simulink subsystem "Vehicle_Model_Simplified"  (R2023b)
settings: Solver=VariableStepAuto  StartTime=0.0  StopTime=10.0  RelTol=1e-3
values from neighbouring files (symbols this model uses):
  phi = 45    [Data_Parse_Events.m]
  theta = Digital_Signals.Corner_Dynamics_Sensors.theta.Data    [Yaw_Tables.m]    (also in compute_axis_transformation.m = acos(dot(XYZs,XYZv)/(norm(XYZv)^2)); create_yaw_table.m = acos(dot(XYZs,XYZv)/(norm(XYZv)^2)))
undefined symbols (not defined in the file or in its folder): chassis, dZ, F0z, powertrain, psi, sim, suspension, VEH, X, Xdot, Y, Ydot, Z, Zdot
libraries: vehdynlibtire x10, vehdynlibsuspension x8, autolibutils x5, sharedtransform x5, shared6dof x2, dspstat3 x1, vehdynlibeom x1, vehdynlibtirecommon x1
(part 2 of 6)

== system Vehicle_Model_Simplified/Suspension/MacPherson Suspension ==
  Wheel : Inport
  Steering : Inport  Port=2
  Vehicle : Inport  Port=3
  Bus Creator1 : BusCreator  Inputs=6
  Bus Creator2 : BusCreator  Inputs=2
  Bus Creator3 : BusCreator  Inputs=2
  Bus Creator4 : BusCreator  Inputs=6
  Bus Selector : BusSelector  OutputSignals=z,Re,zdot,Fx,Fy,M
  Bus Selector1 : BusSelector  OutputSignals=P,V
  Bus Selector2 : BusSelector  OutputSignals=SuspFrame.z
  Selector1 : Selector  NumberOfDimensions=2  IndexOptions=Index vector (dialog),Select all  Indices=1,1  OutputSizes=1,1
  Selector2 : Selector  NumberOfDimensions=2  IndexOptions=Index vector (dialog),Select all  Indices=2,1  OutputSizes=1,1
  Steer Rate Adapter : Subsystem
  Steering Adapter : Subsystem
  Terminator : Terminator
  Terminator1 : Terminator
  Vehicle Adapter : Subsystem
  Wheel  Adapter : Subsystem
  Wheel1 : InportShadow
  independent Suspensions - MacPherson : vehdynlibsuspension/Independent Suspension - MacPherson  ActiveDampEn=off  NumAxl=2  NumWhlsByAxl=[2 2]  StrgEnByAxl=[1 0]  AntiSwayEnByAxl=[1 0]  WhlNumVec="[1  2  1  2]"  AxleNumVec="[1  1  2  2]"  SuspTypesByAxle="[1  1]"  SuspImage=suspmacp.png  IdealSuspEn=on  IdealSuspAxles="[1  2]"  Kz=Kz  F0z=F0z  Cz=Cz  Hmax=Hmax  f_act_susp_cz=[10000 10000;10000 10000]  f_act_susp_duty_bpt=[0 1]  f_act_susp_zdot_bpt=[-1 1]  Toe=0.  RollStrgSlp=0.  ToeStrgSlp=0.  Caster=0.  CasterHslp=0.  CasterStrgSlp=0.  Camber=0.  CamberHslp=0.  CamberStrgSlp=0.  StrgHgtSlp=0.1432  MappedSuspEn=off  MappedSuspAxles="[1  2]"  f_susp_axl_bp=[1 2]  f_susp_dz_bp=[-0.15 -0.14 -0.13 -0.12 -0.11 -0.10 -0.09 -0.08 -0.07 -0.06 -0.05 -0.04 -0.03 -0.02 -0.01 0.00 0.01 0.02 0.03 0.04 0.05 0.06 0.07 0.08 0.09 0.10 0.11 0.12 0.13 0.14 0.15]  f_susp_dzdot_bp=[-0.15 -0.14 -0.13 -0.12 -0.11 -0.10 -0.09 -0.08 -0.07 -0.06 -0.05 -0.04 -0.03 -0.02 -0.01 0.00 0.01 0.02 0.03 0.04 0.05 0.06 0.07 0.08 0.09 0.10 0.11 0.12 0.13 0.14 0.15]  f_susp_fmz=zeros(31,31,61,2,4)  f_susp_geom=zeros(31,61,2,3)  f_susp_strgdelta_bp=[-30,-29,-28,-27,-26,-25,-24,-23,-22,-21,-20,-19,-18,-17,-16,-15,-14,-13,-12,-11,-10,-9,-8,-7,-6,-5,-4,-3,-2,-1,0,1,2,3,4,5,6,7,8,9,10,11,12,13,14,15,16,17,18,19,20,21,22,23,24,25,26,27,28,29,30]  AntiSwayR=0.2  AntiSwayNtrlAng=0.5236  AntiSwayTrsK=8e+02
  Suspension : Outport  VectorParamsAs1DForOutWhenUnconnected=off
  wires:
  Bus Creator3/1 -> Suspension/1
  Bus Creator1/1 -> Bus Creator3/2  "Whl"
  Bus Selector1/2 -> independent Suspensions - MacPherson/8  "<V>"
  Bus Selector/6 -> independent Suspensions - MacPherson/6  "<M>"
  Bus Selector/5 -> independent Suspensions - MacPherson/5  "<Fy>"
  Steering/1 -> Steering Adapter/1(Steer)
  Bus Selector/3 -> independent Suspensions - MacPherson/3  "<zdot>"
  Bus Selector/4 -> independent Suspensions - MacPherson/4  "<Fx>"
  Vehicle/1 -> Vehicle Adapter/1(Veh), Steer Rate Adapter/1(Veh)
  Vehicle Adapter/1(VehSusp) -> Bus Selector1/1
  independent Suspensions - MacPherson/3 -> Bus Creator2/2  "M"
  Wheel  Adapter/2(WhlFy) -> Bus Creator4/2  "Fy"
  Wheel  Adapter/1(WhlFx) -> Bus Creator4/1  "Fx"
  Wheel/1 -> Wheel  Adapter/1(Wheels)
  Wheel  Adapter/3(z) -> Bus Creator4/3
  Wheel  Adapter/4(zdot) -> Bus Creator4/4
  Wheel  Adapter/5(M) -> Bus Creator4/5  "M"
  Wheel  Adapter/6(Re) -> Bus Creator4/6
  Bus Selector/2 -> independent Suspensions - MacPherson/2  "<Re>"
  Selector1/1 -> Bus Creator1/2  "xdot"
  Selector2/1 -> Bus Creator1/3  "ydot"
  Bus Selector1/1 -> independent Suspensions - MacPherson/7  "<P>"
  Bus Selector/1 -> independent Suspensions - MacPherson/1  "<z>"
  independent Suspensions - MacPherson/4 -> Bus Creator1/1  "F"
  independent Suspensions - MacPherson/6 -> Bus Creator1/4  "Ang"
  Vehicle Adapter/2(VehVbody) -> Selector1/1, Selector2/1  "V"
  independent Suspensions - MacPherson/2 -> Bus Creator2/1  "F"
  Bus Creator2/1 -> Bus Creator3/1  "Veh"
  Bus Creator4/1 -> Bus Selector/1
  Steer Rate Adapter/1(AngVel) -> Bus Creator1/6  "AngVel"
  Steering Adapter/1(StrgAng) -> independent Suspensions - MacPherson/9
  independent Suspensions - MacPherson/1 -> Terminator/1
  independent Suspensions - MacPherson/5 -> Terminator1/1  "V"
  Bus Selector2/1 -> Bus Creator1/5  "<z>"
  Wheel1/1 -> Bus Selector2/1

== system Vehicle_Model_Simplified/Suspension/Mapped Suspension ==
  Wheel : Inport
  Steering : Inport  Port=2
  Vehicle : Inport  Port=3
  Bus Creator1 : BusCreator  Inputs=6
  Bus Creator2 : BusCreator  Inputs=2
  Bus Creator3 : BusCreator  Inputs=2
  Bus Creator4 : BusCreator  Inputs=6
  Bus Selector : BusSelector  OutputSignals=z,Re,zdot,Fx,Fy,M
  Bus Selector1 : BusSelector  OutputSignals=P,V
  Bus Selector2 : BusSelector  OutputSignals=SuspFrame.z
  Independent Suspension - Mapped : vehdynlibsuspension/Independent Suspension - Mapped  NumAxl=2  NumWhlsByAxl=[2 2]  StrgEnByAxl=[1 0]  AntiSwayEnByAxl=[1 1]  WhlNumVec="[1  2  1  2]"  AxleNumVec="[1  1  2  2]"  SuspTypesByAxle="[2  2]"  SuspImage=suspindmap.png  IdealSuspEn=off  IdealSuspAxles="[1  2]"  Kz=64370  F0z=9810  Cz=10000  Hmax=0.5  Toe=2  RollStrgSlp=-13  ToeStrgSlp=0.01  Caster=4  CasterHslp=-13  CasterStrgSlp=0.01  Camber=4  CamberHslp=-13  CamberStrgSlp=0.01  StrgHgtSlp=0.0025  MappedSuspEn=on  MappedSuspAxles="[1  2]"  f_susp_axl_bp=[1 2]  f_susp_dz_bp=f_susp_dz_bp  f_susp_dzdot_bp=f_susp_dzdot_bp  f_susp_fmz=f_susp_fmz  f_susp_geom=f_susp_geom  f_susp_strgdelta_bp=f_susp_strgdelta_bp  NDFLookupOutType=1:4  NDGLookupOutType=1:3  AntiSwayR=0.2  AntiSwayNtrlAng=0.5236  AntiSwayTrsK=8e2
      link override For each track and axle combination calculate suspension forces and moments/Suspension/Suspension Angle Calculations: OverrideUsingVariant=MappedSteeringEnabled
      link override For each track and axle combination calculate suspension forces and moments/Suspension/Z axis suspension characteristic: OverrideUsingVariant=MappedSuspension
  Reshape1 : Reshape  OutputDimensionality=Row vector (2-D)
  Selector : Selector  IndexOptions=Index vector (dialog)  Indices=[1 2]  OutputSizes=1
  Selector1 : Selector  NumberOfDimensions=2  IndexOptions=Index vector (dialog),Select all  Indices=1,1  OutputSizes=1,1
  Selector2 : Selector  NumberOfDimensions=2  IndexOptions=Index vector (dialog),Select all  Indices=2,1  OutputSizes=1,1
  Steer Rate Adapter : Subsystem
  Terminator : Terminator
  Terminator1 : Terminator
  Vehicle Adapter : Subsystem
  Wheel  Adapter : Subsystem
  Wheel1 : InportShadow
  Suspension : Outport  VectorParamsAs1DForOutWhenUnconnected=off
  wires:
  Independent Suspension - Mapped/1 -> Terminator/1
  Reshape1/1 -> Independent Suspension - Mapped/9
  Bus Selector/5 -> Independent Suspension - Mapped/5  "<Fy>"
  Bus Selector/2 -> Independent Suspension - Mapped/2  "<Re>"
  Bus Selector1/2 -> Independent Suspension - Mapped/8  "<V>"
  Bus Selector/4 -> Independent Suspension - Mapped/4  "<Fx>"
  Wheel  Adapter/5(M) -> Bus Creator4/5
  Bus Selector/6 -> Independent Suspension - Mapped/6  "<M>"
  Wheel  Adapter/4(zdot) -> Bus Creator4/4
  Wheel  Adapter/6(Re) -> Bus Creator4/6
  Selector/1 -> Reshape1/1
  Bus Creator4/1 -> Bus Selector/1
  Wheel  Adapter/3(z) -> Bus Creator4/3
  Wheel  Adapter/2(WhlFy) -> Bus Creator4/2  "Fy"
  Wheel/1 -> Wheel  Adapter/1(Wheels)
  Vehicle Adapter/1(VehSusp) -> Bus Selector1/1
  Bus Selector/3 -> Independent Suspension - Mapped/3  "<zdot>"
  Bus Selector/1 -> Independent Suspension - Mapped/1  "<z>"
  Wheel  Adapter/1(WhlFx) -> Bus Creator4/1  "Fx"
  Bus Selector1/1 -> Independent Suspension - Mapped/7  "<P>"
  Steering/1 -> Selector/1
  Vehicle/1 -> Vehicle Adapter/1(Veh), Steer Rate Adapter/1(Veh)
  Independent Suspension - Mapped/6 -> Bus Creator1/4  "Ang"
  Selector2/1 -> Bus Creator1/3  "ydot"
  Independent Suspension - Mapped/2 -> Bus Creator2/1  "F"
  Independent Suspension - Mapped/3 -> Bus Creator2/2  "M"
  Bus Creator2/1 -> Bus Creator3/1  "Veh"
  Bus Creator1/1 -> Bus Creator3/2  "Whl"
  Independent Suspension - Mapped/4 -> Bus Creator1/1  "F"
  Selector1/1 -> Bus Creator1/2  "xdot"
  Vehicle Adapter/2(VehVbody) -> Selector1/1, Selector2/1  "V"
  Bus Creator3/1 -> Suspension/1
  Steer Rate Adapter/1(AngVel) -> Bus Creator1/6
  Independent Suspension - Mapped/5 -> Terminator1/1  "V"
  Bus Selector2/1 -> Bus Creator1/5  "<z>"
  Wheel1/1 -> Bus Selector2/1

== system Vehicle_Model_Simplified/Vehicle/6DOF ==
  Suspension : Inport
  Wind : Inport  Port=2
  Constant1 : Constant  Value=[0;0;0]
  Suspension to Chasiss Transforms : Subsystem
  Terminator{,1..5} (6 alike) : Terminator
  Vehicle Body 6DOF : vehdynlibeom/Vehicle Body 6DOF  extPos=on  extVel=on  extEuler=on  extRotRate=on  htchFMode=off  htchMMode=off  m=chassis.mass.m_body+chassis.mass.m_driver  a=chassis.geometry.l(1)  b=chassis.geometry.l(2)  d=0  h=chassis.geometry.dZ  dh=1  hl=0  hh=0.1  Xe_o=[1 1 1].*sim.IC.pos_IC  xbdot_o=sim.IC.vel_IC  eul_o=[1 1 1].*sim.IC.ang_IC  p_o=[1 1 1].*sim.IC.ang_vel_IC  Iveh=chassis.mass.Iveh  w=2.*chassis.geometry.s  z1m=0  z1R=[-.25,.125,.15]  z1I=[1.4,-.2,.1;-.2,1.4,.1;.1,.1,2.25].*0  z2m=0  z2R=[1.4,0,.8]  z2I=[1.4,-.2,.1;-.2,1.4,.1;.1,.1,2.25].*0  z3m=0  z3R=[.75,-.5,.4]  z3I=[5,-.1,-2;-2,9,.1;-.1,.1,6].*0  z4m=0  z4R=[.75,.5,.4]  z4I=[5,-.1,-2;-2,9,.1;-.1,.1,6].*0  z5m=0  z5R=[1.25,-.5,.4]  z5I=[5,-.1,-2;-2,9,.1;-.1,.1,6].*0  z6m=0  z6R=[1.25,-.5,.4]  z6I=[5,-.1,-2;-2,9,.1;-.1,.1,6].*0  z7m=0  z7R=[2,0,.25]  z7I=[1.4,-.2,.1;-.2,1.4,.1;.1,.1,2.25].*0  Af=chassis.aero.Af  Cd=chassis.aero.Cd  Cl=0  Cpm=sim.strange_parameters.cpm  beta_w=sim.strange_parameters.beta_w  Cs=sim.strange_parameters.Cs  Cym=sim.strange_parameters.Cym  Pabs=sim.constant.Pair  extTamb=off  Tair=sim.constant.Tair  g=sim.constant.g  xdot_tol=sim.strange_parameters.xdot_tol  longOff=0  latOff=0  vertOff=0.0112  wrapAng=off  aMode=2
  VehFdbk : Outport  VectorParamsAs1DForOutWhenUnconnected=off
  wires:
  Wind/1 -> Vehicle Body 6DOF/5
  Vehicle Body 6DOF/1 -> VehFdbk/1, Suspension to Chasiss Transforms/1(VehFdbk)  "VehFdbk"
  Constant1/1 -> Vehicle Body 6DOF/4
  Vehicle Body 6DOF/2 -> Terminator/1
  Vehicle Body 6DOF/3 -> Terminator1/1
  Vehicle Body 6DOF/4 -> Terminator2/1
  Vehicle Body 6DOF/5 -> Terminator3/1
  Vehicle Body 6DOF/6 -> Terminator4/1
  Vehicle Body 6DOF/7 -> Terminator5/1
  Suspension/1 -> Suspension to Chasiss Transforms/2(Suspension)
  Suspension to Chasiss Transforms/1(FsB) -> Vehicle Body 6DOF/1
  Suspension to Chasiss Transforms/3(Fext) -> Vehicle Body 6DOF/3
  Suspension to Chasiss Transforms/2(MsB) -> Vehicle Body 6DOF/2

== system Vehicle_Model_Simplified/Wheels and Tires/VDBS ==
  WhlAng : Inport
  WhlCmb : Inport  Port=2  Unit=rad
  AxleTrq : Inport  Port=3
  BrkPed : Inport  Port=4
  Fz : Inport  Port=5  Unit=N
  r : Inport  Port=6
  VehVel : Inport  Port=7
  Ground Level : Inport  Port=8
  Friction : Inport  Port=9  Unit=1  PortDimensions=4
  Veh : Inport  Port=10
  Pressure : vehdynlibtirecommon/Constant  const=82700  numWheels=4
  Terminator : Terminator
  Tire2Veh : Subsystem
  Tires : Subsystem  Variant=on  VariantControlMode=label  VariantControl=Variant1  LabelModeActiveChoice=2
  Veh2Tire : Subsystem
  scale factors with friction : Subsystem  mask{numWheels=4}
      mask prompts: numWheels "Number of wheels"
  Wheels : Outport  VectorParamsAs1DForOutWhenUnconnected=off
  Wheels2Susp : Outport  Port=2  VectorParamsAs1DForOutWhenUnconnected=off
  FrntAxlF : Outport  Port=3  Unit=N  VectorParamsAs1DForOutWhenUnconnected=off
  RearAxlF : Outport  Port=4  Unit=N  VectorParamsAs1DForOutWhenUnconnected=off
  Omega : Outport  Port=5  VectorParamsAs1DForOutWhenUnconnected=off
  Mz : Outport  Port=6  Unit=N*m  VectorParamsAs1DForOutWhenUnconnected=off
  SuspWhlPz : Outport  Port=7  VectorParamsAs1DForOutWhenUnconnected=off
  SuspWhlVz : Outport  Port=8  VectorParamsAs1DForOutWhenUnconnected=off
  wires:
  Ground Level/1 -> Tires/9("Gnd ")
  Pressure/1 -> Tires/7("Press ")
  scale factors with friction/1(lambdas) -> Tires/8("lambda ")
  Fz/1 -> Tire2Veh/3(Fz), Tires/10("FzSusp ")
  AxleTrq/1 -> Veh2Tire/2(Axle)
  BrkPed/1 -> Veh2Tire/3(Brake Pedal)
  VehVel/1 -> Veh2Tire/4(VehVel)
  Veh2Tire/1(T) -> Tires/1("DriveTorque ")
  Veh2Tire/2(P) -> Tires/2(Brake Pedal)
  Veh2Tire/4(xdotAxle) -> Tires/4("Vx ")
  Veh2Tire/5(ydotAxle) -> Tires/5("Vy ")
  Veh2Tire/3(psidot) -> Tires/3("r ")
  WhlAng/1 -> Veh2Tire/5(WhlAng), Tire2Veh/5(WhlAng)
  Tire2Veh/3(Omega) -> Omega/1
  Tire2Veh/4(FrntAxlF) -> FrntAxlF/1
  Tire2Veh/5(RearAxlF) -> RearAxlF/1
  Tire2Veh/6(<Mz>) -> Mz/1
  Friction/1 -> scale factors with friction/2(lamda_mu_y), scale factors with friction/1(lamda_mu_x)
  r/1 -> Veh2Tire/1(r)
  Veh2Tire/6(zdotAxle) -> Terminator/1
  Tire2Veh/7(SuspWhlPz) -> SuspWhlPz/1
  Tire2Veh/8(SuspWhlVz) -> SuspWhlVz/1
  Veh/1 -> Tire2Veh/1(Veh)
  Tire2Veh/2(Wheels2Susp) -> Wheels2Susp/1
  Tires/1(" Wheels") -> Tire2Veh/2(Wheels)  "TireFrame"
  Tire2Veh/1(Wheel) -> Wheels/1
  WhlCmb/1 -> Tire2Veh/4(WhlCmb), Veh2Tire/6(WhlCmb)  "WhlCamberIn"
  Veh2Tire/7(Camber) -> Tires/6("Camber ")

== system Vehicle_Model_Simplified/Suspension/Double Wishbone Suspension/Steer Rate Adapter ==
  Veh : Inport
  Add : Sum
  Bus Selector3 : BusSelector  OutputSignals=BdyFrm.Cg.AngVel.r
  Constant : Constant  Value=zeros(1,4)
  Matrix Concatenate : Concatenate  NumInputs=3  Mode=Multidimensional array
  Matrix Concatenate1 : Concatenate  NumInputs=3  Mode=Multidimensional array
  Reshape2 : Reshape  OutputDimensionality=Row vector (2-D)
  Reshape3 : Reshape  OutputDimensionality=Row vector (2-D)
  Reshape4 : Reshape  OutputDimensionality=Row vector (2-D)
  Selector3 : Selector  InputPortWidth=1  IndexOptions=Index vector (dialog)  Indices=[1 1 1 1]  OutputSizes=1
  SteerRates : Constant  Value=zeros(1,4)
  AngVel : Outport  VectorParamsAs1DForOutWhenUnconnected=off
  wires:
  Reshape2/1 -> Matrix Concatenate1/1, Matrix Concatenate1/3, Matrix Concatenate1/2
  Constant/1 -> Reshape3/1
  Selector3/1 -> Reshape4/1
  Bus Selector3/1 -> Selector3/1  "<r>"
  Matrix Concatenate/1 -> Add/2
  SteerRates/1 -> Reshape2/1
  Reshape4/1 -> Matrix Concatenate/3
  Reshape3/1 -> Matrix Concatenate/2, Matrix Concatenate/1
  Matrix Concatenate1/1 -> Add/1
  Veh/1 -> Bus Selector3/1
  Add/1 -> AngVel/1  "AngVel"

== system Vehicle_Model_Simplified/Suspension/Double Wishbone Suspension/Steering Adapter ==
  Steer : Inport
  Reshape1 : Reshape  OutputDimensionality=Row vector (2-D)
  Selector : Selector  IndexOptions=Index vector (dialog)  Indices=[1 2]  OutputSizes=1
  Steering Model : Subsystem
  StrgAng : Outport  VectorParamsAs1DForOutWhenUnconnected=off
  wires:
  Reshape1/1 -> StrgAng/1
  Selector/1 -> Reshape1/1
  Steering Model/1(steering_angles) -> Selector/1
  Steer/1 -> Steering Model/1(steering_angle)

== system Vehicle_Model_Simplified/Suspension/Double Wishbone Suspension/Vehicle Adapter ==
  Veh : Inport
  Bus Creator3 : BusCreator  Inputs=2
  Bus Selector1 : BusSelector  OutputSignals=InertFrm.FrntAxl.Lft.Disp.X,InertFrm.FrntAxl.Lft.Disp.Y,InertFrm.FrntAxl.Lft.Disp.Z,InertFrm.FrntAxl.Rght.Disp.X,InertFrm.FrntAxl.Rght.Disp.Y,InertFrm.FrntAxl.Rght.Disp.Z,InertFrm.RearAxl.Lft.Disp.X,InertFrm.RearAxl.Lft.Disp.Y,InertFrm.RearAxl.Lft.Disp.Z,InertFrm.RearAxl.Rght.Disp.X,InertFrm.RearAxl.Rght.Disp.Y,InertFrm.RearAxl.Rght.Disp.Z
  Bus Selector2 : BusSelector  OutputSignals=BdyFrm.FrntAxl.Lft.Vel.xdot,BdyFrm.FrntAxl.Lft.Vel.ydot,BdyFrm.FrntAxl.Lft.Vel.zdot,BdyFrm.FrntAxl.Rght.Vel.xdot,BdyFrm.FrntAxl.Rght.Vel.ydot,BdyFrm.FrntAxl.Rght.Vel.zdot,BdyFrm.RearAxl.Lft.Vel.xdot,BdyFrm.RearAxl.Lft.Vel.ydot,BdyFrm.RearAxl.Lft.Vel.zdot,BdyFrm.RearAxl.Rght.Vel.xdot,BdyFrm.RearAxl.Rght.Vel.ydot,BdyFrm.RearAxl.Rght.Vel.zdot
  Bus Selector3 : BusSelector  OutputSignals=InertFrm.FrntAxl.Lft.Vel.Xdot,InertFrm.FrntAxl.Lft.Vel.Ydot,InertFrm.FrntAxl.Lft.Vel.Zdot,InertFrm.FrntAxl.Rght.Vel.Xdot,InertFrm.FrntAxl.Rght.Vel.Ydot,InertFrm.FrntAxl.Rght.Vel.Zdot,InertFrm.RearAxl.Lft.Vel.Xdot,InertFrm.RearAxl.Lft.Vel.Ydot,InertFrm.RearAxl.Lft.Vel.Zdot,InertFrm.RearAxl.Rght.Vel.Xdot,InertFrm.RearAxl.Rght.Vel.Ydot,InertFrm.RearAxl.Rght.Vel.Zdot
  Inertial Frame CG to Axle Offset : Constant  Value=[zeros(2,4);chassis.geometry.dZ*ones(1,4)]
  Mux1 : Mux  Inputs=12
  Mux2 : Mux  Inputs=12
  Mux3 : Mux  Inputs=12
  Reshape : Reshape  OutputDimensionality=Customize  OutputDimensions=[3,4]
  Reshape1 : Reshape  OutputDimensionality=Customize  OutputDimensions=[3,4]
  Reshape2 : Reshape  OutputDimensionality=Customize  OutputDimensions=[3,4]
  Sum : Sum  Inputs=|+-
  VehSusp : Outport  VectorParamsAs1DForOutWhenUnconnected=off
  VehVbody : Outport  Port=2  VectorParamsAs1DForOutWhenUnconnected=off
  wires:
  Veh/1 -> Bus Selector3/1, Bus Selector2/1, Bus Selector1/1
  Reshape2/1 -> VehVbody/1  "V"
  Bus Creator3/1 -> VehSusp/1  "Veh"
  Reshape/1 -> Sum/1
  Bus Selector1/1 -> Mux2/1  "<X>"
  Bus Selector1/2 -> Mux2/2  "<Y>"
  Bus Selector1/3 -> Mux2/3  "<Z>"
  Bus Selector1/4 -> Mux2/4  "<X>"
  Bus Selector1/5 -> Mux2/5  "<Y>"
  Bus Selector1/6 -> Mux2/6  "<Z>"
  Bus Selector1/7 -> Mux2/7  "<X>"
  Bus Selector1/8 -> Mux2/8  "<Y>"
  Bus Selector1/9 -> Mux2/9  "<Z>"
  Bus Selector1/10 -> Mux2/10  "<X>"
  Bus Selector1/11 -> Mux2/11  "<Y>"
  Bus Selector1/12 -> Mux2/12  "<Z>"
  Bus Selector2/1 -> Mux1/1  "<xdot>"
  Bus Selector2/2 -> Mux1/2  "<ydot>"
  Bus Selector2/3 -> Mux1/3  "<zdot>"
  Bus Selector2/4 -> Mux1/4  "<xdot>"
  Bus Selector2/5 -> Mux1/5  "<ydot>"
  Bus Selector2/6 -> Mux1/6  "<zdot>"
  Bus Selector2/7 -> Mux1/7  "<xdot>"
  Bus Selector2/8 -> Mux1/8  "<ydot>"
  Bus Selector2/9 -> Mux1/9  "<zdot>"
  Bus Selector2/10 -> Mux1/10  "<xdot>"
  Bus Selector2/11 -> Mux1/11  "<ydot>"
  Bus Selector2/12 -> Mux1/12  "<zdot>"
  Mux1/1 -> Reshape2/1
  Mux2/1 -> Reshape/1
  Inertial Frame CG to Axle Offset/1 -> Sum/2
  Sum/1 -> Bus Creator3/1  "P"
  Mux3/1 -> Reshape1/1
  Bus Selector3/12 -> Mux3/12  "<Zdot>"
  Bus Selector3/11 -> Mux3/11  "<Ydot>"
  Bus Selector3/10 -> Mux3/10  "<Xdot>"
  Bus Selector3/9 -> Mux3/9  "<Zdot>"
  Bus Selector3/8 -> Mux3/8  "<Ydot>"
  Bus Selector3/7 -> Mux3/7  "<Xdot>"
  Bus Selector3/6 -> Mux3/6  "<Zdot>"
  Bus Selector3/5 -> Mux3/5  "<Ydot>"
  Bus Selector3/4 -> Mux3/4  "<Xdot>"
  Bus Selector3/3 -> Mux3/3  "<Zdot>"
  Bus Selector3/2 -> Mux3/2  "<Ydot>"
  Bus Selector3/1 -> Mux3/1  "<Xdot>"
  Reshape1/1 -> Bus Creator3/2  "V"

== system Vehicle_Model_Simplified/Suspension/Double Wishbone Suspension/Wheel  Adapter ==
  Wheels : Inport
  Bus Selector : BusSelector  OutputSignals=SuspFrame.Fx,SuspFrame.Fy
  Bus Selector1 : BusSelector  OutputSignals=SuspFrame.Re
  Bus Selector2 : BusSelector  OutputSignals=SuspFrame.Mx,SuspFrame.My,SuspFrame.Mz
  Bus Selector3 : BusSelector  OutputSignals=SuspFrame.z,SuspFrame.zdot
  Matrix Concatenate : Concatenate  NumInputs=3  Mode=Multidimensional array
  Reshape{,1..7} (8 alike) : Reshape  OutputDimensionality=Row vector (2-D)
  WhlFx : Outport  VectorParamsAs1DForOutWhenUnconnected=off
  WhlFy : Outport  Port=2  VectorParamsAs1DForOutWhenUnconnected=off
  z : Outport  Port=3  VectorParamsAs1DForOutWhenUnconnected=off
  zdot : Outport  Port=4  VectorParamsAs1DForOutWhenUnconnected=off
  M : Outport  Port=5  VectorParamsAs1DForOutWhenUnconnected=off
  Re : Outport  Port=6  VectorParamsAs1DForOutWhenUnconnected=off
  wires:
  Reshape7/1 -> WhlFy/1
  Reshape6/1 -> WhlFx/1
  Bus Selector/1 -> Reshape6/1  "<Fx>"
  Bus Selector/2 -> Reshape7/1  "<Fy>"
  Bus Selector3/1 -> Reshape/1  "<z>"
  Wheels/1 -> Bus Selector1/1, Bus Selector2/1, Bus Selector3/1, Bus Selector/1
  Bus Selector3/2 -> Reshape2/1  "<zdot>"
  Reshape2/1 -> zdot/1  "zdot"
  Bus Selector1/1 -> Reshape1/1  "<Re>"
  Reshape1/1 -> Re/1  "Re"
  Bus Selector2/1 -> Reshape3/1  "<Mx>"
  Bus Selector2/2 -> Reshape4/1  "<My>"
  Bus Selector2/3 -> Reshape5/1  "<Mz>"
  Reshape3/1 -> Matrix Concatenate/1
  Reshape4/1 -> Matrix Concatenate/2
  Reshape5/1 -> Matrix Concatenate/3
  Matrix Concatenate/1 -> M/1  "M"
  Reshape/1 -> z/1  "z"

== system Vehicle_Model_Simplified/Suspension/Independent Mapped Front Suspension Mapped Solid Axle Rear Suspension/Steer Rate Adapter ==
  Veh : Inport
  Add : Sum
  Bus Selector3 : BusSelector  OutputSignals=BdyFrm.Cg.AngVel.r
  Constant : Constant  Value=zeros(1,4)
  Matrix Concatenate : Concatenate  NumInputs=3  Mode=Multidimensional array
  Matrix Concatenate1 : Concatenate  NumInputs=3  Mode=Multidimensional array
  Reshape2 : Reshape  OutputDimensionality=Row vector (2-D)
  Reshape3 : Reshape  OutputDimensionality=Row vector (2-D)
  Reshape4 : Reshape  OutputDimensionality=Row vector (2-D)
  Selector3 : Selector  InputPortWidth=1  IndexOptions=Index vector (dialog)  Indices=[1 1 1 1]  OutputSizes=1
  SteerRates : Constant  Value=zeros(1,4)
  AngVel : Outport  VectorParamsAs1DForOutWhenUnconnected=off
  wires:
  Reshape2/1 -> Matrix Concatenate1/1, Matrix Concatenate1/3, Matrix Concatenate1/2
  Constant/1 -> Reshape3/1
  Selector3/1 -> Reshape4/1
  Bus Selector3/1 -> Selector3/1  "<r>"
  Matrix Concatenate/1 -> Add/2
  SteerRates/1 -> Reshape2/1
  Reshape4/1 -> Matrix Concatenate/3
  Reshape3/1 -> Matrix Concatenate/2, Matrix Concatenate/1
  Matrix Concatenate1/1 -> Add/1
  Veh/1 -> Bus Selector3/1
  Add/1 -> AngVel/1  "AngVel"

== system Vehicle_Model_Simplified/Suspension/Independent Mapped Front Suspension Mapped Solid Axle Rear Suspension/Steering Adapter ==
  Steer : Inport
  Reshape1 : Reshape  OutputDimensionality=Row vector (2-D)
  Selector : Selector  IndexOptions=Index vector (dialog)  Indices=[1 2]  OutputSizes=1
  StrgAng : Outport  VectorParamsAs1DForOutWhenUnconnected=off
  wires:
  Reshape1/1 -> StrgAng/1
  Steer/1 -> Selector/1
  Selector/1 -> Reshape1/1

== system Vehicle_Model_Simplified/Suspension/Independent Mapped Front Suspension Mapped Solid Axle Rear Suspension/Vehicle Adapter ==
  Veh : Inport
  Bus Creator3 : BusCreator  Inputs=2
  Bus Selector1 : BusSelector  OutputSignals=InertFrm.FrntAxl.Lft.Disp.X,InertFrm.FrntAxl.Lft.Disp.Y,InertFrm.FrntAxl.Lft.Disp.Z,InertFrm.FrntAxl.Rght.Disp.X,InertFrm.FrntAxl.Rght.Disp.Y,InertFrm.FrntAxl.Rght.Disp.Z,InertFrm.RearAxl.Lft.Disp.X,InertFrm.RearAxl.Lft.Disp.Y,InertFrm.RearAxl.Lft.Disp.Z,InertFrm.RearAxl.Rght.Disp.X,InertFrm.RearAxl.Rght.Disp.Y,InertFrm.RearAxl.Rght.Disp.Z
  Bus Selector2 : BusSelector  OutputSignals=BdyFrm.FrntAxl.Lft.Vel.xdot,BdyFrm.FrntAxl.Lft.Vel.ydot,BdyFrm.FrntAxl.Lft.Vel.zdot,BdyFrm.FrntAxl.Rght.Vel.xdot,BdyFrm.FrntAxl.Rght.Vel.ydot,BdyFrm.FrntAxl.Rght.Vel.zdot,BdyFrm.RearAxl.Lft.Vel.xdot,BdyFrm.RearAxl.Lft.Vel.ydot,BdyFrm.RearAxl.Lft.Vel.zdot,BdyFrm.RearAxl.Rght.Vel.xdot,BdyFrm.RearAxl.Rght.Vel.ydot,BdyFrm.RearAxl.Rght.Vel.zdot
  Bus Selector3 : BusSelector  OutputSignals=InertFrm.FrntAxl.Lft.Vel.Xdot,InertFrm.FrntAxl.Lft.Vel.Ydot,InertFrm.FrntAxl.Lft.Vel.Zdot,InertFrm.FrntAxl.Rght.Vel.Xdot,InertFrm.FrntAxl.Rght.Vel.Ydot,InertFrm.FrntAxl.Rght.Vel.Zdot,InertFrm.RearAxl.Lft.Vel.Xdot,InertFrm.RearAxl.Lft.Vel.Ydot,InertFrm.RearAxl.Lft.Vel.Zdot,InertFrm.RearAxl.Rght.Vel.Xdot,InertFrm.RearAxl.Rght.Vel.Ydot,InertFrm.RearAxl.Rght.Vel.Zdot
  Inertial Frame CG to Axle Offset : Constant  Value=[zeros(2,4);VEH.HeightCG*ones(1,4)]
  Mux1 : Mux  Inputs=12
  Mux2 : Mux  Inputs=12
  Mux3 : Mux  Inputs=12
  Reshape : Reshape  OutputDimensionality=Customize  OutputDimensions=[3,4]
  Reshape1 : Reshape  OutputDimensionality=Customize  OutputDimensions=[3,4]
  Reshape2 : Reshape  OutputDimensionality=Customize  OutputDimensions=[3,4]
  Sum : Sum  Inputs=|+-
  VehSusp : Outport  VectorParamsAs1DForOutWhenUnconnected=off
  VehVbody : Outport  Port=2  VectorParamsAs1DForOutWhenUnconnected=off
  wires:
  Veh/1 -> Bus Selector3/1, Bus Selector2/1, Bus Selector1/1
  Reshape2/1 -> VehVbody/1  "V"
  Bus Creator3/1 -> VehSusp/1  "Veh"
  Reshape/1 -> Sum/1
  Bus Selector1/1 -> Mux2/1  "<X>"
  Bus Selector1/2 -> Mux2/2  "<Y>"
  Bus Selector1/3 -> Mux2/3  "<Z>"
  Bus Selector1/4 -> Mux2/4  "<X>"
  Bus Selector1/5 -> Mux2/5  "<Y>"
  Bus Selector1/6 -> Mux2/6  "<Z>"
  Bus Selector1/7 -> Mux2/7  "<X>"
  Bus Selector1/8 -> Mux2/8  "<Y>"
  Bus Selector1/9 -> Mux2/9  "<Z>"
  Bus Selector1/10 -> Mux2/10  "<X>"
  Bus Selector1/11 -> Mux2/11  "<Y>"
  Bus Selector1/12 -> Mux2/12  "<Z>"
  Bus Selector2/1 -> Mux1/1  "<xdot>"
  Bus Selector2/2 -> Mux1/2  "<ydot>"
  Bus Selector2/3 -> Mux1/3  "<zdot>"
  Bus Selector2/4 -> Mux1/4  "<xdot>"
  Bus Selector2/5 -> Mux1/5  "<ydot>"
  Bus Selector2/6 -> Mux1/6  "<zdot>"
  Bus Selector2/7 -> Mux1/7  "<xdot>"
  Bus Selector2/8 -> Mux1/8  "<ydot>"
  Bus Selector2/9 -> Mux1/9  "<zdot>"
  Bus Selector2/10 -> Mux1/10  "<xdot>"
  Bus Selector2/11 -> Mux1/11  "<ydot>"
  Bus Selector2/12 -> Mux1/12  "<zdot>"
  Mux1/1 -> Reshape2/1
  Mux2/1 -> Reshape/1
  Inertial Frame CG to Axle Offset/1 -> Sum/2
  Sum/1 -> Bus Creator3/1  "P"
  Mux3/1 -> Reshape1/1
  Bus Selector3/12 -> Mux3/12  "<Zdot>"
  Bus Selector3/11 -> Mux3/11  "<Ydot>"
  Bus Selector3/10 -> Mux3/10  "<Xdot>"
  Bus Selector3/9 -> Mux3/9  "<Zdot>"
  Bus Selector3/8 -> Mux3/8  "<Ydot>"
  Bus Selector3/7 -> Mux3/7  "<Xdot>"
  Bus Selector3/6 -> Mux3/6  "<Zdot>"
  Bus Selector3/5 -> Mux3/5  "<Ydot>"
  Bus Selector3/4 -> Mux3/4  "<Xdot>"
  Bus Selector3/3 -> Mux3/3  "<Zdot>"
  Bus Selector3/2 -> Mux3/2  "<Ydot>"
  Bus Selector3/1 -> Mux3/1  "<Xdot>"
  Reshape1/1 -> Bus Creator3/2  "V"

== system Vehicle_Model_Simplified/Suspension/Independent Mapped Front Suspension Mapped Solid Axle Rear Suspension/Wheel  Adapter ==
  Wheels : Inport
  Bus Selector : BusSelector  OutputSignals=SuspFrame.Fx,SuspFrame.Fy
  Bus Selector1 : BusSelector  OutputSignals=SuspFrame.Re
  Bus Selector2 : BusSelector  OutputSignals=SuspFrame.Mx,SuspFrame.My,SuspFrame.Mz
  Bus Selector3 : BusSelector  OutputSignals=SuspFrame.z,SuspFrame.zdot
  Matrix Concatenate : Concatenate  NumInputs=3  Mode=Multidimensional array
  Reshape{,1..7} (8 alike) : Reshape  OutputDimensionality=Row vector (2-D)
  WhlFx : Outport  VectorParamsAs1DForOutWhenUnconnected=off
  WhlFy : Outport  Port=2  VectorParamsAs1DForOutWhenUnconnected=off
  z : Outport  Port=3  VectorParamsAs1DForOutWhenUnconnected=off
  zdot : Outport  Port=4  VectorParamsAs1DForOutWhenUnconnected=off
  M : Outport  Port=5  VectorParamsAs1DForOutWhenUnconnected=off
  Re : Outport  Port=6  VectorParamsAs1DForOutWhenUnconnected=off
  wires:
  Reshape7/1 -> WhlFy/1
  Reshape6/1 -> WhlFx/1
  Bus Selector/1 -> Reshape6/1  "<Fx>"
  Bus Selector/2 -> Reshape7/1  "<Fy>"
  Bus Selector3/1 -> Reshape/1  "<z>"
  Wheels/1 -> Bus Selector1/1, Bus Selector2/1, Bus Selector3/1, Bus Selector/1
  Bus Selector3/2 -> Reshape2/1  "<zdot>"
  Reshape2/1 -> zdot/1  "zdot"
  Bus Selector1/1 -> Reshape1/1  "<Re>"
  Reshape1/1 -> Re/1  "Re"
  Bus Selector2/1 -> Reshape3/1  "<Mx>"
  Bus Selector2/2 -> Reshape4/1  "<My>"
  Bus Selector2/3 -> Reshape5/1  "<Mz>"
  Reshape3/1 -> Matrix Concatenate/1
  Reshape4/1 -> Matrix Concatenate/2
  Reshape5/1 -> Matrix Concatenate/3
  Matrix Concatenate/1 -> M/1  "M"
  Reshape/1 -> z/1  "z"

== system Vehicle_Model_Simplified/Suspension/Kinematics and Compliance Independent Suspension/Calculate dynamic track width from lateral wheel center displacement change ==
  dWhlY : Inport
  dWhlZ : Inport  Port=2
  Front Track Calculation : Subsystem
  Gain : Gain  Gain=-1
  Rear Track Calculation : Subsystem
  Sign : Signum  ZeroCross=off
  Vector Concatenate : Concatenate
  w : Outport
  wires:
  dWhlZ/1 -> Gain/1
  dWhlY/1 -> Rear Track Calculation/1(dWhlY), Front Track Calculation/1(dWhlY)
  Vector Concatenate/1 -> w/1
  Front Track Calculation/1(w_front) -> Vector Concatenate/1
  Rear Track Calculation/1(w_rear) -> Vector Concatenate/2
  Sign/1 -> Rear Track Calculation/2(sign), Front Track Calculation/2(sign)
  Gain/1 -> Sign/1

== system Vehicle_Model_Simplified/Suspension/Kinematics and Compliance Independent Suspension/Steer Rate Adapter ==
  Veh : Inport
  Add : Sum
  Bus Selector3 : BusSelector  OutputSignals=BdyFrm.Cg.AngVel.r
  Constant : Constant  Value=zeros(1,4)
  Matrix Concatenate : Concatenate  NumInputs=3  Mode=Multidimensional array
  Matrix Concatenate1 : Concatenate  NumInputs=3  Mode=Multidimensional array
  Reshape2 : Reshape  OutputDimensionality=Row vector (2-D)
  Reshape3 : Reshape  OutputDimensionality=Row vector (2-D)
  Reshape4 : Reshape  OutputDimensionality=Row vector (2-D)
  Selector3 : Selector  InputPortWidth=1  IndexOptions=Index vector (dialog)  Indices=[1 1 1 1]  OutputSizes=1
  SteerRates : Constant  Value=zeros(1,4)
  AngVel : Outport  VectorParamsAs1DForOutWhenUnconnected=off
  wires:
  Reshape2/1 -> Matrix Concatenate1/1, Matrix Concatenate1/3, Matrix Concatenate1/2
  Constant/1 -> Reshape3/1
  Selector3/1 -> Reshape4/1
  Bus Selector3/1 -> Selector3/1  "<r>"
  Matrix Concatenate/1 -> Add/2
  SteerRates/1 -> Reshape2/1
  Reshape4/1 -> Matrix Concatenate/3
  Reshape3/1 -> Matrix Concatenate/2, Matrix Concatenate/1
  Matrix Concatenate1/1 -> Add/1
  Veh/1 -> Bus Selector3/1
  Add/1 -> AngVel/1  "AngVel"

== system Vehicle_Model_Simplified/Suspension/Kinematics and Compliance Independent Suspension/Steering Adapter ==
  Steer : Inport
  Reshape1 : Reshape  OutputDimensionality=Row vector (2-D)
  Selector : Selector  IndexOptions=Index vector (dialog)  Indices=[1 2]  OutputSizes=1
  StrgAng : Outport  VectorParamsAs1DForOutWhenUnconnected=off
  wires:
  Reshape1/1 -> StrgAng/1
  Steer/1 -> Selector/1
  Selector/1 -> Reshape1/1

== system Vehicle_Model_Simplified/Suspension/Kinematics and Compliance Independent Suspension/Vehicle Adapter ==
  Veh : Inport
  Bus Creator3 : BusCreator  Inputs=2
  Bus Selector1 : BusSelector  OutputSignals=InertFrm.FrntAxl.Lft.Disp.X,InertFrm.FrntAxl.Lft.Disp.Y,InertFrm.FrntAxl.Lft.Disp.Z,InertFrm.FrntAxl.Rght.Disp.X,InertFrm.FrntAxl.Rght.Disp.Y,InertFrm.FrntAxl.Rght.Disp.Z,InertFrm.RearAxl.Lft.Disp.X,InertFrm.RearAxl.Lft.Disp.Y,InertFrm.RearAxl.Lft.Disp.Z,InertFrm.RearAxl.Rght.Disp.X,InertFrm.RearAxl.Rght.Disp.Y,InertFrm.RearAxl.Rght.Disp.Z
  Bus Selector2 : BusSelector  OutputSignals=BdyFrm.FrntAxl.Lft.Vel.xdot,BdyFrm.FrntAxl.Lft.Vel.ydot,BdyFrm.FrntAxl.Lft.Vel.zdot,BdyFrm.FrntAxl.Rght.Vel.xdot,BdyFrm.FrntAxl.Rght.Vel.ydot,BdyFrm.FrntAxl.Rght.Vel.zdot,BdyFrm.RearAxl.Lft.Vel.xdot,BdyFrm.RearAxl.Lft.Vel.ydot,BdyFrm.RearAxl.Lft.Vel.zdot,BdyFrm.RearAxl.Rght.Vel.xdot,BdyFrm.RearAxl.Rght.Vel.ydot,BdyFrm.RearAxl.Rght.Vel.zdot
  Bus Selector3 : BusSelector  OutputSignals=InertFrm.FrntAxl.Lft.Vel.Xdot,InertFrm.FrntAxl.Lft.Vel.Ydot,InertFrm.FrntAxl.Lft.Vel.Zdot,InertFrm.FrntAxl.Rght.Vel.Xdot,InertFrm.FrntAxl.Rght.Vel.Ydot,InertFrm.FrntAxl.Rght.Vel.Zdot,InertFrm.RearAxl.Lft.Vel.Xdot,InertFrm.RearAxl.Lft.Vel.Ydot,InertFrm.RearAxl.Lft.Vel.Zdot,InertFrm.RearAxl.Rght.Vel.Xdot,InertFrm.RearAxl.Rght.Vel.Ydot,InertFrm.RearAxl.Rght.Vel.Zdot
  Inertial Frame CG to Axle Offset : Constant  Value=[zeros(2,4);VEH.HeightCG*ones(1,4)]
  Mux1 : Mux  Inputs=12
  Mux2 : Mux  Inputs=12
  Mux3 : Mux  Inputs=12
  Reshape : Reshape  OutputDimensionality=Customize  OutputDimensions=[3,4]
  Reshape1 : Reshape  OutputDimensionality=Customize  OutputDimensions=[3,4]
  Reshape2 : Reshape  OutputDimensionality=Customize  OutputDimensions=[3,4]
  Sum : Sum  Inputs=|+-
  VehSusp : Outport  VectorParamsAs1DForOutWhenUnconnected=off
  VehVbody : Outport  Port=2  VectorParamsAs1DForOutWhenUnconnected=off
  wires:
  Veh/1 -> Bus Selector3/1, Bus Selector2/1, Bus Selector1/1
  Reshape2/1 -> VehVbody/1  "V"
  Bus Creator3/1 -> VehSusp/1  "Veh"
  Reshape/1 -> Sum/1
  Bus Selector1/1 -> Mux2/1  "<X>"
  Bus Selector1/2 -> Mux2/2  "<Y>"
  Bus Selector1/3 -> Mux2/3  "<Z>"
  Bus Selector1/4 -> Mux2/4  "<X>"
  Bus Selector1/5 -> Mux2/5  "<Y>"
  Bus Selector1/6 -> Mux2/6  "<Z>"
  Bus Selector1/7 -> Mux2/7  "<X>"
  Bus Selector1/8 -> Mux2/8  "<Y>"
  Bus Selector1/9 -> Mux2/9  "<Z>"
  Bus Selector1/10 -> Mux2/10  "<X>"
  Bus Selector1/11 -> Mux2/11  "<Y>"
  Bus Selector1/12 -> Mux2/12  "<Z>"
  Bus Selector2/1 -> Mux1/1  "<xdot>"
  Bus Selector2/2 -> Mux1/2  "<ydot>"
  Bus Selector2/3 -> Mux1/3  "<zdot>"
  Bus Selector2/4 -> Mux1/4  "<xdot>"
  Bus Selector2/5 -> Mux1/5  "<ydot>"
  Bus Selector2/6 -> Mux1/6  "<zdot>"
  Bus Selector2/7 -> Mux1/7  "<xdot>"
  Bus Selector2/8 -> Mux1/8  "<ydot>"
  Bus Selector2/9 -> Mux1/9  "<zdot>"
  Bus Selector2/10 -> Mux1/10  "<xdot>"
  Bus Selector2/11 -> Mux1/11  "<ydot>"
  Bus Selector2/12 -> Mux1/12  "<zdot>"
  Mux1/1 -> Reshape2/1
  Mux2/1 -> Reshape/1
  Inertial Frame CG to Axle Offset/1 -> Sum/2
  Sum/1 -> Bus Creator3/1  "P"
  Mux3/1 -> Reshape1/1
  Bus Selector3/12 -> Mux3/12  "<Zdot>"
  Bus Selector3/11 -> Mux3/11  "<Ydot>"
  Bus Selector3/10 -> Mux3/10  "<Xdot>"
  Bus Selector3/9 -> Mux3/9  "<Zdot>"
  Bus Selector3/8 -> Mux3/8  "<Ydot>"
  Bus Selector3/7 -> Mux3/7  "<Xdot>"
  Bus Selector3/6 -> Mux3/6  "<Zdot>"
  Bus Selector3/5 -> Mux3/5  "<Ydot>"
  Bus Selector3/4 -> Mux3/4  "<Xdot>"
  Bus Selector3/3 -> Mux3/3  "<Zdot>"
  Bus Selector3/2 -> Mux3/2  "<Ydot>"
  Bus Selector3/1 -> Mux3/1  "<Xdot>"
  Reshape1/1 -> Bus Creator3/2  "V"

== system Vehicle_Model_Simplified/Suspension/Kinematics and Compliance Independent Suspension/Wheel  Adapter ==
  Wheels : Inport
  Bus Selector : BusSelector  OutputSignals=SuspFrame.Fx,SuspFrame.Fy
  Bus Selector1 : BusSelector  OutputSignals=SuspFrame.Re
  Bus Selector2 : BusSelector  OutputSignals=SuspFrame.Mx,SuspFrame.My,SuspFrame.Mz
  Bus Selector3 : BusSelector  OutputSignals=SuspFrame.z,SuspFrame.zdot
  Matrix Concatenate : Concatenate  NumInputs=3  Mode=Multidimensional array
  Reshape{,1..7} (8 alike) : Reshape  OutputDimensionality=Row vector (2-D)
  WhlFx : Outport  VectorParamsAs1DForOutWhenUnconnected=off
  WhlFy : Outport  Port=2  VectorParamsAs1DForOutWhenUnconnected=off
  z : Outport  Port=3  VectorParamsAs1DForOutWhenUnconnected=off
  zdot : Outport  Port=4  VectorParamsAs1DForOutWhenUnconnected=off
  M : Outport  Port=5  VectorParamsAs1DForOutWhenUnconnected=off
  Re : Outport  Port=6  VectorParamsAs1DForOutWhenUnconnected=off
  wires:
  Reshape7/1 -> WhlFy/1
  Reshape6/1 -> WhlFx/1
  Bus Selector/1 -> Reshape6/1  "<Fx>"
  Bus Selector/2 -> Reshape7/1  "<Fy>"
  Bus Selector3/1 -> Reshape/1  "<z>"
  Wheels/1 -> Bus Selector1/1, Bus Selector2/1, Bus Selector3/1, Bus Selector/1
  Bus Selector3/2 -> Reshape2/1  "<zdot>"
  Reshape2/1 -> zdot/1  "zdot"
  Bus Selector1/1 -> Reshape1/1  "<Re>"
  Reshape1/1 -> Re/1  "Re"
  Bus Selector2/1 -> Reshape3/1  "<Mx>"
  Bus Selector2/2 -> Reshape4/1  "<My>"
  Bus Selector2/3 -> Reshape5/1  "<Mz>"
  Reshape3/1 -> Matrix Concatenate/1
  Reshape4/1 -> Matrix Concatenate/2
  Reshape5/1 -> Matrix Concatenate/3
  Matrix Concatenate/1 -> M/1  "M"
  Reshape/1 -> z/1  "z"

== system Vehicle_Model_Simplified/Suspension/MacPherson Front Suspension Solid Axle Rear Suspension/Steer Rate Adapter ==
  Veh : Inport
  Add : Sum
  Bus Selector3 : BusSelector  OutputSignals=BdyFrm.Cg.AngVel.r
  Constant : Constant  Value=zeros(1,4)
  Matrix Concatenate : Concatenate  NumInputs=3  Mode=Multidimensional array
  Matrix Concatenate1 : Concatenate  NumInputs=3  Mode=Multidimensional array
  Reshape2 : Reshape  OutputDimensionality=Row vector (2-D)
  Reshape3 : Reshape  OutputDimensionality=Row vector (2-D)
  Reshape4 : Reshape  OutputDimensionality=Row vector (2-D)
  Selector3 : Selector  InputPortWidth=1  IndexOptions=Index vector (dialog)  Indices=[1 1 1 1]  OutputSizes=1
  SteerRates : Constant  Value=zeros(1,4)
  AngVel : Outport  VectorParamsAs1DForOutWhenUnconnected=off
  wires:
  Reshape2/1 -> Matrix Concatenate1/1, Matrix Concatenate1/3, Matrix Concatenate1/2
  Constant/1 -> Reshape3/1
  Selector3/1 -> Reshape4/1
  Bus Selector3/1 -> Selector3/1  "<r>"
  Matrix Concatenate/1 -> Add/2
  SteerRates/1 -> Reshape2/1
  Reshape4/1 -> Matrix Concatenate/3
  Reshape3/1 -> Matrix Concatenate/2, Matrix Concatenate/1
  Matrix Concatenate1/1 -> Add/1
  Veh/1 -> Bus Selector3/1
  Add/1 -> AngVel/1  "AngVel"

== system Vehicle_Model_Simplified/Suspension/MacPherson Front Suspension Solid Axle Rear Suspension/Steering Adapter ==
  Steer : Inport
  Reshape1 : Reshape  OutputDimensionality=Row vector (2-D)
  Selector : Selector  IndexOptions=Index vector (dialog)  Indices=[1 2]  OutputSizes=1
  StrgAng : Outport  VectorParamsAs1DForOutWhenUnconnected=off
  wires:
  Reshape1/1 -> StrgAng/1
  Steer/1 -> Selector/1
  Selector/1 -> Reshape1/1

== system Vehicle_Model_Simplified/Suspension/MacPherson Front Suspension Solid Axle Rear Suspension/Vehicle Adapter ==
  Veh : Inport
  Bus Creator3 : BusCreator  Inputs=2
  Bus Selector1 : BusSelector  OutputSignals=InertFrm.FrntAxl.Lft.Disp.X,InertFrm.FrntAxl.Lft.Disp.Y,InertFrm.FrntAxl.Lft.Disp.Z,InertFrm.FrntAxl.Rght.Disp.X,InertFrm.FrntAxl.Rght.Disp.Y,InertFrm.FrntAxl.Rght.Disp.Z,InertFrm.RearAxl.Lft.Disp.X,InertFrm.RearAxl.Lft.Disp.Y,InertFrm.RearAxl.Lft.Disp.Z,InertFrm.RearAxl.Rght.Disp.X,InertFrm.RearAxl.Rght.Disp.Y,InertFrm.RearAxl.Rght.Disp.Z
  Bus Selector2 : BusSelector  OutputSignals=BdyFrm.FrntAxl.Lft.Vel.xdot,BdyFrm.FrntAxl.Lft.Vel.ydot,BdyFrm.FrntAxl.Lft.Vel.zdot,BdyFrm.FrntAxl.Rght.Vel.xdot,BdyFrm.FrntAxl.Rght.Vel.ydot,BdyFrm.FrntAxl.Rght.Vel.zdot,BdyFrm.RearAxl.Lft.Vel.xdot,BdyFrm.RearAxl.Lft.Vel.ydot,BdyFrm.RearAxl.Lft.Vel.zdot,BdyFrm.RearAxl.Rght.Vel.xdot,BdyFrm.RearAxl.Rght.Vel.ydot,BdyFrm.RearAxl.Rght.Vel.zdot
  Bus Selector3 : BusSelector  OutputSignals=InertFrm.FrntAxl.Lft.Vel.Xdot,InertFrm.FrntAxl.Lft.Vel.Ydot,InertFrm.FrntAxl.Lft.Vel.Zdot,InertFrm.FrntAxl.Rght.Vel.Xdot,InertFrm.FrntAxl.Rght.Vel.Ydot,InertFrm.FrntAxl.Rght.Vel.Zdot,InertFrm.RearAxl.Lft.Vel.Xdot,InertFrm.RearAxl.Lft.Vel.Ydot,InertFrm.RearAxl.Lft.Vel.Zdot,InertFrm.RearAxl.Rght.Vel.Xdot,InertFrm.RearAxl.Rght.Vel.Ydot,InertFrm.RearAxl.Rght.Vel.Zdot
  Inertial Frame CG to Axle Offset : Constant  Value=[zeros(2,4);VEH.HeightCG*ones(1,4)]
  Mux1 : Mux  Inputs=12
  Mux2 : Mux  Inputs=12
  Mux3 : Mux  Inputs=12
  Reshape : Reshape  OutputDimensionality=Customize  OutputDimensions=[3,4]
  Reshape1 : Reshape  OutputDimensionality=Customize  OutputDimensions=[3,4]
  Reshape2 : Reshape  OutputDimensionality=Customize  OutputDimensions=[3,4]
  Sum : Sum  Inputs=|+-
  VehSusp : Outport  VectorParamsAs1DForOutWhenUnconnected=off
  VehVbody : Outport  Port=2  VectorParamsAs1DForOutWhenUnconnected=off
  wires:
  Veh/1 -> Bus Selector3/1, Bus Selector2/1, Bus Selector1/1
  Reshape2/1 -> VehVbody/1  "V"
  Bus Creator3/1 -> VehSusp/1  "Veh"
  Reshape/1 -> Sum/1
  Bus Selector1/1 -> Mux2/1  "<X>"
  Bus Selector1/2 -> Mux2/2  "<Y>"
  Bus Selector1/3 -> Mux2/3  "<Z>"
  Bus Selector1/4 -> Mux2/4  "<X>"
  Bus Selector1/5 -> Mux2/5  "<Y>"
  Bus Selector1/6 -> Mux2/6  "<Z>"
  Bus Selector1/7 -> Mux2/7  "<X>"
  Bus Selector1/8 -> Mux2/8  "<Y>"
  Bus Selector1/9 -> Mux2/9  "<Z>"
  Bus Selector1/10 -> Mux2/10  "<X>"
  Bus Selector1/11 -> Mux2/11  "<Y>"
  Bus Selector1/12 -> Mux2/12  "<Z>"
  Bus Selector2/1 -> Mux1/1  "<xdot>"
  Bus Selector2/2 -> Mux1/2  "<ydot>"
  Bus Selector2/3 -> Mux1/3  "<zdot>"
  Bus Selector2/4 -> Mux1/4  "<xdot>"
  Bus Selector2/5 -> Mux1/5  "<ydot>"
  Bus Selector2/6 -> Mux1/6  "<zdot>"
  Bus Selector2/7 -> Mux1/7  "<xdot>"
  Bus Selector2/8 -> Mux1/8  "<ydot>"
  Bus Selector2/9 -> Mux1/9  "<zdot>"
  Bus Selector2/10 -> Mux1/10  "<xdot>"
  Bus Selector2/11 -> Mux1/11  "<ydot>"
  Bus Selector2/12 -> Mux1/12  "<zdot>"
  Mux1/1 -> Reshape2/1
  Mux2/1 -> Reshape/1
  Inertial Frame CG to Axle Offset/1 -> Sum/2
  Sum/1 -> Bus Creator3/1  "P"
  Mux3/1 -> Reshape1/1
  Bus Selector3/12 -> Mux3/12  "<Zdot>"
  Bus Selector3/11 -> Mux3/11  "<Ydot>"
  Bus Selector3/10 -> Mux3/10  "<Xdot>"
  Bus Selector3/9 -> Mux3/9  "<Zdot>"
  Bus Selector3/8 -> Mux3/8  "<Ydot>"
  Bus Selector3/7 -> Mux3/7  "<Xdot>"
  Bus Selector3/6 -> Mux3/6  "<Zdot>"
  Bus Selector3/5 -> Mux3/5  "<Ydot>"
  Bus Selector3/4 -> Mux3/4  "<Xdot>"
  Bus Selector3/3 -> Mux3/3  "<Zdot>"
  Bus Selector3/2 -> Mux3/2  "<Ydot>"
  Bus Selector3/1 -> Mux3/1  "<Xdot>"
  Reshape1/1 -> Bus Creator3/2  "V"

== system Vehicle_Model_Simplified/Suspension/MacPherson Front Suspension Solid Axle Rear Suspension/Wheel  Adapter ==
  Wheels : Inport
  Bus Selector : BusSelector  OutputSignals=SuspFrame.Fx,SuspFrame.Fy
  Bus Selector1 : BusSelector  OutputSignals=SuspFrame.Re
  Bus Selector2 : BusSelector  OutputSignals=SuspFrame.Mx,SuspFrame.My,SuspFrame.Mz
  Bus Selector3 : BusSelector  OutputSignals=SuspFrame.z,SuspFrame.zdot
  Matrix Concatenate : Concatenate  NumInputs=3  Mode=Multidimensional array
  Reshape{,1..7} (8 alike) : Reshape  OutputDimensionality=Row vector (2-D)
  WhlFx : Outport  VectorParamsAs1DForOutWhenUnconnected=off
  WhlFy : Outport  Port=2  VectorParamsAs1DForOutWhenUnconnected=off
  z : Outport  Port=3  VectorParamsAs1DForOutWhenUnconnected=off
  zdot : Outport  Port=4  VectorParamsAs1DForOutWhenUnconnected=off
  M : Outport  Port=5  VectorParamsAs1DForOutWhenUnconnected=off
  Re : Outport  Port=6  VectorParamsAs1DForOutWhenUnconnected=off
  wires:
  Reshape7/1 -> WhlFy/1
  Reshape6/1 -> WhlFx/1
  Bus Selector/1 -> Reshape6/1  "<Fx>"
  Bus Selector/2 -> Reshape7/1  "<Fy>"
  Bus Selector3/1 -> Reshape/1  "<z>"
  Wheels/1 -> Bus Selector1/1, Bus Selector2/1, Bus Selector3/1, Bus Selector/1
  Bus Selector3/2 -> Reshape2/1  "<zdot>"
  Reshape2/1 -> zdot/1  "zdot"
  Bus Selector1/1 -> Reshape1/1  "<Re>"
  Reshape1/1 -> Re/1  "Re"
  Bus Selector2/1 -> Reshape3/1  "<Mx>"
  Bus Selector2/2 -> Reshape4/1  "<My>"
  Bus Selector2/3 -> Reshape5/1  "<Mz>"
  Reshape3/1 -> Matrix Concatenate/1
  Reshape4/1 -> Matrix Concatenate/2
  Reshape5/1 -> Matrix Concatenate/3
  Matrix Concatenate/1 -> M/1  "M"
  Reshape/1 -> z/1  "z"

== system Vehicle_Model_Simplified/Suspension/MacPherson Suspension/Steer Rate Adapter ==
  Veh : Inport
  Add : Sum
  Bus Selector3 : BusSelector  OutputSignals=BdyFrm.Cg.AngVel.r
  Constant : Constant  Value=zeros(1,4)
  Matrix Concatenate : Concatenate  NumInputs=3  Mode=Multidimensional array
  Matrix Concatenate1 : Concatenate  NumInputs=3  Mode=Multidimensional array
  Reshape2 : Reshape  OutputDimensionality=Row vector (2-D)
  Reshape3 : Reshape  OutputDimensionality=Row vector (2-D)
  Reshape4 : Reshape  OutputDimensionality=Row vector (2-D)
  Selector3 : Selector  InputPortWidth=1  IndexOptions=Index vector (dialog)  Indices=[1 1 1 1]  OutputSizes=1
  SteerRates : Constant  Value=zeros(1,4)
  AngVel : Outport  VectorParamsAs1DForOutWhenUnconnected=off
  wires:
  Reshape2/1 -> Matrix Concatenate1/1, Matrix Concatenate1/3, Matrix Concatenate1/2
  Constant/1 -> Reshape3/1
  Selector3/1 -> Reshape4/1
  Bus Selector3/1 -> Selector3/1  "<r>"
  Matrix Concatenate/1 -> Add/2
  SteerRates/1 -> Reshape2/1
  Reshape4/1 -> Matrix Concatenate/3
  Reshape3/1 -> Matrix Concatenate/2, Matrix Concatenate/1
  Matrix Concatenate1/1 -> Add/1
  Veh/1 -> Bus Selector3/1
  Add/1 -> AngVel/1  "AngVel"

== system Vehicle_Model_Simplified/Suspension/MacPherson Suspension/Steering Adapter ==
  Steer : Inport
  Reshape1 : Reshape  OutputDimensionality=Row vector (2-D)
  Selector : Selector  IndexOptions=Index vector (dialog)  Indices=[1 2]  OutputSizes=1
  StrgAng : Outport  VectorParamsAs1DForOutWhenUnconnected=off
  wires:
  Reshape1/1 -> StrgAng/1
  Steer/1 -> Selector/1
  Selector/1 -> Reshape1/1

== system Vehicle_Model_Simplified/Suspension/MacPherson Suspension/Vehicle Adapter ==
  Veh : Inport
  Bus Creator3 : BusCreator  Inputs=2
  Bus Selector1 : BusSelector  OutputSignals=InertFrm.FrntAxl.Lft.Disp.X,InertFrm.FrntAxl.Lft.Disp.Y,InertFrm.FrntAxl.Lft.Disp.Z,InertFrm.FrntAxl.Rght.Disp.X,InertFrm.FrntAxl.Rght.Disp.Y,InertFrm.FrntAxl.Rght.Disp.Z,InertFrm.RearAxl.Lft.Disp.X,InertFrm.RearAxl.Lft.Disp.Y,InertFrm.RearAxl.Lft.Disp.Z,InertFrm.RearAxl.Rght.Disp.X,InertFrm.RearAxl.Rght.Disp.Y,InertFrm.RearAxl.Rght.Disp.Z
  Bus Selector2 : BusSelector  OutputSignals=BdyFrm.FrntAxl.Lft.Vel.xdot,BdyFrm.FrntAxl.Lft.Vel.ydot,BdyFrm.FrntAxl.Lft.Vel.zdot,BdyFrm.FrntAxl.Rght.Vel.xdot,BdyFrm.FrntAxl.Rght.Vel.ydot,BdyFrm.FrntAxl.Rght.Vel.zdot,BdyFrm.RearAxl.Lft.Vel.xdot,BdyFrm.RearAxl.Lft.Vel.ydot,BdyFrm.RearAxl.Lft.Vel.zdot,BdyFrm.RearAxl.Rght.Vel.xdot,BdyFrm.RearAxl.Rght.Vel.ydot,BdyFrm.RearAxl.Rght.Vel.zdot
  Bus Selector3 : BusSelector  OutputSignals=InertFrm.FrntAxl.Lft.Vel.Xdot,InertFrm.FrntAxl.Lft.Vel.Ydot,InertFrm.FrntAxl.Lft.Vel.Zdot,InertFrm.FrntAxl.Rght.Vel.Xdot,InertFrm.FrntAxl.Rght.Vel.Ydot,InertFrm.FrntAxl.Rght.Vel.Zdot,InertFrm.RearAxl.Lft.Vel.Xdot,InertFrm.RearAxl.Lft.Vel.Ydot,InertFrm.RearAxl.Lft.Vel.Zdot,InertFrm.RearAxl.Rght.Vel.Xdot,InertFrm.RearAxl.Rght.Vel.Ydot,InertFrm.RearAxl.Rght.Vel.Zdot
  Inertial Frame CG to Axle Offset : Constant  Value=[zeros(2,4);VEH.HeightCG*ones(1,4)]
  Mux1 : Mux  Inputs=12
  Mux2 : Mux  Inputs=12
  Mux3 : Mux  Inputs=12
  Reshape : Reshape  OutputDimensionality=Customize  OutputDimensions=[3,4]
  Reshape1 : Reshape  OutputDimensionality=Customize  OutputDimensions=[3,4]
  Reshape2 : Reshape  OutputDimensionality=Customize  OutputDimensions=[3,4]
  Sum : Sum  Inputs=|+-
  VehSusp : Outport  VectorParamsAs1DForOutWhenUnconnected=off
  VehVbody : Outport  Port=2  VectorParamsAs1DForOutWhenUnconnected=off
  wires:
  Veh/1 -> Bus Selector3/1, Bus Selector2/1, Bus Selector1/1
  Reshape2/1 -> VehVbody/1  "V"
  Bus Creator3/1 -> VehSusp/1  "Veh"
  Reshape/1 -> Sum/1
  Bus Selector1/1 -> Mux2/1  "<X>"
  Bus Selector1/2 -> Mux2/2  "<Y>"
  Bus Selector1/3 -> Mux2/3  "<Z>"
  Bus Selector1/4 -> Mux2/4  "<X>"
  Bus Selector1/5 -> Mux2/5  "<Y>"
  Bus Selector1/6 -> Mux2/6  "<Z>"
  Bus Selector1/7 -> Mux2/7  "<X>"
  Bus Selector1/8 -> Mux2/8  "<Y>"
  Bus Selector1/9 -> Mux2/9  "<Z>"
  Bus Selector1/10 -> Mux2/10  "<X>"
  Bus Selector1/11 -> Mux2/11  "<Y>"
  Bus Selector1/12 -> Mux2/12  "<Z>"
  Bus Selector2/1 -> Mux1/1  "<xdot>"
  Bus Selector2/2 -> Mux1/2  "<ydot>"
  Bus Selector2/3 -> Mux1/3  "<zdot>"
  Bus Selector2/4 -> Mux1/4  "<xdot>"
  Bus Selector2/5 -> Mux1/5  "<ydot>"
  Bus Selector2/6 -> Mux1/6  "<zdot>"
  Bus Selector2/7 -> Mux1/7  "<xdot>"
  Bus Selector2/8 -> Mux1/8  "<ydot>"
  Bus Selector2/9 -> Mux1/9  "<zdot>"
  Bus Selector2/10 -> Mux1/10  "<xdot>"
  Bus Selector2/11 -> Mux1/11  "<ydot>"
  Bus Selector2/12 -> Mux1/12  "<zdot>"
  Mux1/1 -> Reshape2/1
  Mux2/1 -> Reshape/1
  Inertial Frame CG to Axle Offset/1 -> Sum/2
  Sum/1 -> Bus Creator3/1  "P"
  Mux3/1 -> Reshape1/1
  Bus Selector3/12 -> Mux3/12  "<Zdot>"
  Bus Selector3/11 -> Mux3/11  "<Ydot>"
  Bus Selector3/10 -> Mux3/10  "<Xdot>"
  Bus Selector3/9 -> Mux3/9  "<Zdot>"
  Bus Selector3/8 -> Mux3/8  "<Ydot>"
  Bus Selector3/7 -> Mux3/7  "<Xdot>"
  Bus Selector3/6 -> Mux3/6  "<Zdot>"
  Bus Selector3/5 -> Mux3/5  "<Ydot>"
  Bus Selector3/4 -> Mux3/4  "<Xdot>"
  Bus Selector3/3 -> Mux3/3  "<Zdot>"
  Bus Selector3/2 -> Mux3/2  "<Ydot>"
  Bus Selector3/1 -> Mux3/1  "<Xdot>"
  Reshape1/1 -> Bus Creator3/2  "V"

== system Vehicle_Model_Simplified/Suspension/MacPherson Suspension/Wheel  Adapter ==
  Wheels : Inport
  Bus Selector : BusSelector  OutputSignals=SuspFrame.Fx,SuspFrame.Fy
  Bus Selector1 : BusSelector  OutputSignals=SuspFrame.Re
  Bus Selector2 : BusSelector  OutputSignals=SuspFrame.Mx,SuspFrame.My,SuspFrame.Mz
  Bus Selector3 : BusSelector  OutputSignals=SuspFrame.z,SuspFrame.zdot
  Matrix Concatenate : Concatenate  NumInputs=3  Mode=Multidimensional array
  Reshape{,1..7} (8 alike) : Reshape  OutputDimensionality=Row vector (2-D)
  WhlFx : Outport  VectorParamsAs1DForOutWhenUnconnected=off
  WhlFy : Outport  Port=2  VectorParamsAs1DForOutWhenUnconnected=off
  z : Outport  Port=3  VectorParamsAs1DForOutWhenUnconnected=off
  zdot : Outport  Port=4  VectorParamsAs1DForOutWhenUnconnected=off
  M : Outport  Port=5  VectorParamsAs1DForOutWhenUnconnected=off
  Re : Outport  Port=6  VectorParamsAs1DForOutWhenUnconnected=off
  wires:
  Reshape7/1 -> WhlFy/1
  Reshape6/1 -> WhlFx/1
  Bus Selector/1 -> Reshape6/1  "<Fx>"
  Bus Selector/2 -> Reshape7/1  "<Fy>"
  Bus Selector3/1 -> Reshape/1  "<z>"
  Wheels/1 -> Bus Selector1/1, Bus Selector2/1, Bus Selector3/1, Bus Selector/1
  Bus Selector3/2 -> Reshape2/1  "<zdot>"
  Reshape2/1 -> zdot/1  "zdot"
  Bus Selector1/1 -> Reshape1/1  "<Re>"
  Reshape1/1 -> Re/1  "Re"
  Bus Selector2/1 -> Reshape3/1  "<Mx>"
  Bus Selector2/2 -> Reshape4/1  "<My>"
  Bus Selector2/3 -> Reshape5/1  "<Mz>"
  Reshape3/1 -> Matrix Concatenate/1
  Reshape4/1 -> Matrix Concatenate/2
  Reshape5/1 -> Matrix Concatenate/3
  Matrix Concatenate/1 -> M/1  "M"
  Reshape/1 -> z/1  "z"
